simulink model "mrefrobotarm_previous_y_previous_u_previous_ref_cex_3b"  (R2018b)
settings: Solver=FixedStepAuto  StartTime=0.0  StopTime=20  RelTol=1e-3  AbsTol=1e-6
undefined symbols (not defined in the file or in its folder): cc, options
libraries: neural x462, simulink x2
(part 12 of 18)

== system mrefrobotarm_previous_y_previous_u_previous_ref_cex_3b/cex_m1/Layer 3/Delays 1 ==
  "p{3}" : Inport  PortDimensions=30
      mask Display: e = 0.06;c1 = [120 230 180]/255;c2 = ([120 230 180]+0)/(256+128);c3 = ([120 230 180]+128)/(256+128);patch([0 1 1 0],[0 0 1 1],c1);patch([0 1 1 1-e 1-e 0+e],[0 0 1 1-e 0+e 0+e],c2);patch([0 0 1 1-e 0+e 0+e],[0 1 1 1-e 1-e 0+e],c3);plot([0 1 1 0 0],[0 0 1 1 0]);
  mux : Mux  Inputs=1
      mask Display: e = 0.06;c1 = [120 150 230]/255;c2 = ([120 150 230]+0)/383;c3 = ([120 150 230]+128)/383;patch([0 1 1 0],[0 0 1 1],c1);patch([0 1 1 1-e 1-e 0+e],[0 0 1 1-e 0+e 0+e],c2);patch([0 0 1 1-e 0+e 0+e],[0 1 1 1-e 1-e 0+e],c3);plot([0 1 1 0 0],[0 0 1 1 0]);disp('Mux')
  "pd{3,2}" : Outport
      mask Display: e = 0.06;c1 = [120 230 180]/255;c2 = ([120 230 180]+0)/(256+128);c3 = ([120 230 180]+128)/(256+128);patch([0 1 1 0],[0 0 1 1],c1);patch([0 1 1 1-e 1-e 0+e],[0 0 1 1-e 0+e 0+e],c2);patch([0 0 1 1-e 0+e 0+e],[0 1 1 1-e 1-e 0+e],c3);plot([0 1 1 0 0],[0 0 1 1 0]);
  wires:
  "p{3}"/1 -> mux/1
  mux/1 -> "pd{3,2}"/1

== system mrefrobotarm_previous_y_previous_u_previous_ref_cex_3b/cex_m1/Layer 3/LW{3,2} ==
  "ad{3,2}" : Inport  PortDimensions=30
      mask Display: e = 0.06;c1 = [120 230 180]/255;c2 = ([120 230 180]+0)/(256+128);c3 = ([120 230 180]+128)/(256+128);patch([0 1 1 0],[0 0 1 1],c1);patch([0 1 1 1-e 1-e 0+e],[0 0 1 1-e 0+e 0+e],c2);patch([0 0 1 1-e 0+e 0+e],[0 1 1 1-e 1-e 0+e],c3);plot([0 1 1 0 0],[0 0 1 1 0]);
  "IW{3,2}(1,:)'" : Constant  Value=[0.0255900601227965381057050109347983379848301410675048828125;-0.2445332719523497233549136353758512996137142181396484375;0.2132234013283009488315400403735111467540264129638671875;-0.0515001036072283702171858976726070977747440338134765625;-0.19351367720373280345569355631596408784389495849609375;0.376109267327173701911391390240169130265712738037109375;0.0666749128615344577308832185735809616744518280029296875;-0.44077680308893107952172840668936260044574737548828125;-0.1774770708842355604328844265182851813733577728271484375;-0.054251675677824177934649441112924250774085521697998046875;0.407756480058180159620206950421561487019062042236328125;-0.11043832971419904886989371561867301352322101593017578125;-0.06656652324338363513334115850739181041717529296875;-0.309772314576237606242870015194057486951351165771484375;-0.2782579958208721837564780798857100307941436767578125;0.0014079282704737897634339471863995640887878835201263427734375;0.164750395979450681149813817683025263249874114990234375;0.03374371873575258973243506943617830984294414520263671875;-0.11697430223199604959471997744913096539676189422607421875;-0.377976875689660485324594674239051528275012969970703125;0.180234815360957700836053163584438152611255645751953125;0.049494338029175431736828016937579377554357051849365234375;-0.541724329864333054018743496271781623363494873046875;0.70957921545389057715880198884406127035617828369140625;-0.2236538006543592749242321815472678281366825103759765625;-0.0168625825253284934712727505257134907878935337066650390625;-0.061157151815638820246956441906149848364293575286865234375;0.0962999458349639014809184800469665788114070892333984375;-0.195422183072548050208894210300059057772159576416015625;0.469008564925858462135721538288635201752185821533203125]
      mask Display: e = 0.06;c1 = [120 150 230]/255;c2 = ([120 150 230]+0)/383;c3 = ([120 150 230]+128)/383;patch([0 1 1 0],[0 0 1 1],c1);patch([0 1 1 1-e 1-e 0+e],[0 0 1 1-e 0+e 0+e],c2);patch([0 0 1 1-e 0+e 0+e],[0 1 1 1-e 1-e 0+e],c3);plot([0 1 1 0 0],[0 0 1 1 0]);disp('weights');
  Mux : Mux  Inputs=1
      mask Display: e = 0.06;c1 = [120 150 230]/255;c2 = ([120 150 230]+0)/383;c3 = ([120 150 230]+128)/383;patch([0 1 1 0],[0 0 1 1],c1);patch([0 1 1 1-e 1-e 0+e],[0 0 1 1-e 0+e 0+e],c2);patch([0 0 1 1-e 0+e 0+e],[0 1 1 1-e 1-e 0+e],c3);plot([0 1 1 0 0],[0 0 1 1 0]);disp('Mux');
  dotprod1 : neural/Weight Functions/dotprod
  "lz{3,2}" : Outport
      mask Display: e = 0.06;c1 = [120 230 180]/255;c2 = ([120 230 180]+0)/(256+128);c3 = ([120 230 180]+128)/(256+128);patch([0 1 1 0],[0 0 1 1],c1);patch([0 1 1 1-e 1-e 0+e],[0 0 1 1-e 0+e 0+e],c2);patch([0 0 1 1-e 0+e 0+e],[0 1 1 1-e 1-e 0+e],c3);plot([0 1 1 0 0],[0 0 1 1 0]);
  wires:
  "IW{3,2}(1,:)'"/1 -> dotprod1/1
  "ad{3,2}"/1 -> dotprod1/2
  dotprod1/1 -> Mux/1
  Mux/1 -> "lz{3,2}"/1

== system mrefrobotarm_previous_y_previous_u_previous_ref_cex_3b/cex_m5/Layer 1/Delays 1 ==
  "p{1}" : Inport  PortDimensions=10
      mask Display: e = 0.06;c1 = [120 230 180]/255;c2 = ([120 230 180]+0)/(256+128);c3 = ([120 230 180]+128)/(256+128);patch([0 1 1 0],[0 0 1 1],c1);patch([0 1 1 1-e 1-e 0+e],[0 0 1 1-e 0+e 0+e],c2);patch([0 0 1 1-e 0+e 0+e],[0 1 1 1-e 1-e 0+e],c3);plot([0 1 1 0 0],[0 0 1 1 0]);
  mux : Mux  Inputs=1
      mask Display: e = 0.06;c1 = [120 150 230]/255;c2 = ([120 150 230]+0)/383;c3 = ([120 150 230]+128)/383;patch([0 1 1 0],[0 0 1 1],c1);patch([0 1 1 1-e 1-e 0+e],[0 0 1 1-e 0+e 0+e],c2);patch([0 0 1 1-e 0+e 0+e],[0 1 1 1-e 1-e 0+e],c3);plot([0 1 1 0 0],[0 0 1 1 0]);disp('Mux')
  "pd{1,1}" : Outport
      mask Display: e = 0.06;c1 = [120 230 180]/255;c2 = ([120 230 180]+0)/(256+128);c3 = ([120 230 180]+128)/(256+128);patch([0 1 1 0],[0 0 1 1],c1);patch([0 1 1 1-e 1-e 0+e],[0 0 1 1-e 0+e 0+e],c2);patch([0 0 1 1-e 0+e 0+e],[0 1 1 1-e 1-e 0+e],c3);plot([0 1 1 0 0],[0 0 1 1 0]);
  wires:
  "p{1}"/1 -> mux/1
  mux/1 -> "pd{1,1}"/1

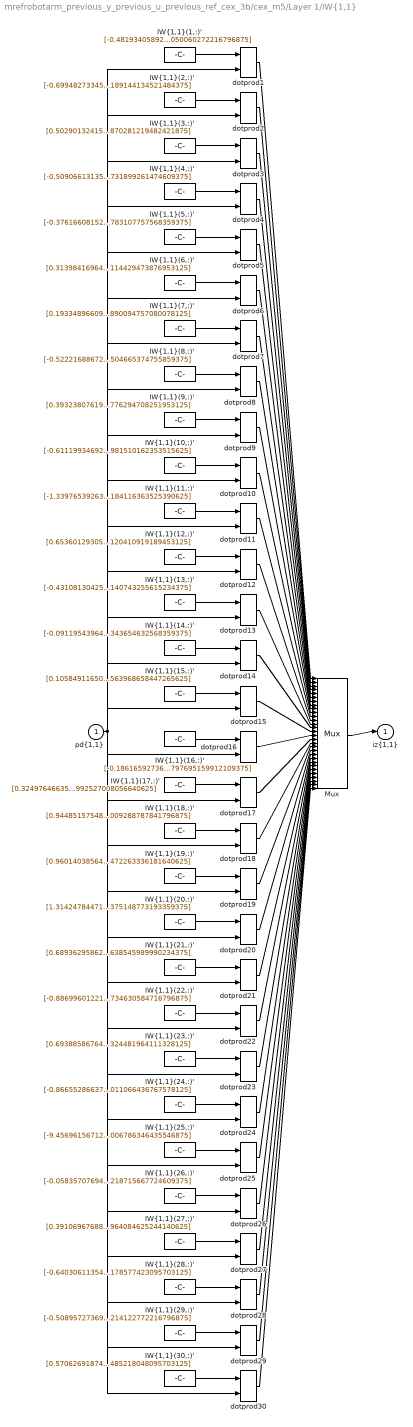
== system mrefrobotarm_previous_y_previous_u_previous_ref_cex_3b/cex_m5/Layer 1/IW{1,1} ==
  "pd{1,1}" : Inport  PortDimensions=10
      mask Display: e = 0.06;c1 = [120 230 180]/255;c2 = ([120 230 180]+0)/(256+128);c3 = ([120 230 180]+128)/(256+128);patch([0 1 1 0],[0 0 1 1],c1);patch([0 1 1 1-e 1-e 0+e],[0 0 1 1-e 0+e 0+e],c2);patch([0 0 1 1-e 0+e 0+e],[0 1 1 1-e 1-e 0+e],c3);plot([0 1 1 0 0],[0 0 1 1 0]);
  "IW{1,1}(1,:)'" : Constant  Value=[-0.481934058923276398278545684661366976797580718994140625;0.36530523689031058065523893674253486096858978271484375;-0.86926905168321899619598980279988609254360198974609375;-0.422931186541281534108094319890369661152362823486328125;0.50571230197535843586820192285813391208648681640625;-0.51255895275061913451963846455328166484832763671875;0.2023427088065134216154916657615103758871555328369140625;0.725871649925782680412567060557194054126739501953125;-0.16849060637558366249066921227495186030864715576171875;-0.205273588229551495754066081644850783050060272216796875]
      mask Display: e = 0.06;c1 = [120 150 230]/255;c2 = ([120 150 230]+0)/383;c3 = ([120 150 230]+128)/383;patch([0 1 1 0],[0 0 1 1],c1);patch([0 1 1 1-e 1-e 0+e],[0 0 1 1-e 0+e 0+e],c2);patch([0 0 1 1-e 0+e 0+e],[0 1 1 1-e 1-e 0+e],c3);plot([0 1 1 0 0],[0 0 1 1 0]);disp('Weights');
  "IW{1,1}(10,:)'" : Constant  Value=[-0.61119934692369726203509117112844251096248626708984375;0.70454804335546794558098326888284645974636077880859375;0.057135643818077175293268510358757339417934417724609375;0.89228683122494256707568638375960290431976318359375;-0.306202450351405086603762129016104154288768768310546875;-0.53945258802536877329458775420789606869220733642578125;0.413295177296751081730263877034303732216358184814453125;-0.86207965190394852950106496791704557836055755615234375;-0.77818630476135786100400082432315684854984283447265625;-0.9866456915733705645976669984520412981510162353515625]
      mask Display: e = 0.06;c1 = [120 150 230]/255;c2 = ([120 150 230]+0)/383;c3 = ([120 150 230]+128)/383;patch([0 1 1 0],[0 0 1 1],c1);patch([0 1 1 1-e 1-e 0+e],[0 0 1 1-e 0+e 0+e],c2);patch([0 0 1 1-e 0+e 0+e],[0 1 1 1-e 1-e 0+e],c3);plot([0 1 1 0 0],[0 0 1 1 0]);disp('Weights');
  "IW{1,1}(11,:)'" : Constant  Value=[-1.3397653926357528941792907062335871160030364990234375;2.106003584289421137754061419400386512279510498046875;-1.3291512443981907676260334483231417834758758544921875;0.462989686404331413083212964920676313340663909912109375;-6.6943247779396433116971820709295570850372314453125;0.1574200960671499893717140139415278099477291107177734375;3.689170060642462001254671122296713292598724365234375;0.455374095081902907633519816954503767192363739013671875;-3.653332928797798473397051566280424594879150390625;-2.427542355801075135701694307499565184116363525390625]
      mask Display: e = 0.06;c1 = [120 150 230]/255;c2 = ([120 150 230]+0)/383;c3 = ([120 150 230]+128)/383;patch([0 1 1 0],[0 0 1 1],c1);patch([0 1 1 1-e 1-e 0+e],[0 0 1 1-e 0+e 0+e],c2);patch([0 0 1 1-e 0+e 0+e],[0 1 1 1-e 1-e 0+e],c3);plot([0 1 1 0 0],[0 0 1 1 0]);disp('Weights');
  "IW{1,1}(12,:)'" : Constant  Value=[0.6536012930577299595569229495595209300518035888671875;-0.9465981615866529974567811223096214234828948974609375;0.68180864552264408562365360921830870211124420166015625;0.95131511966430759574819830959313549101352691650390625;-0.63476802573249646588493533272412605583667755126953125;0.51713095973796685544954243596293963491916656494140625;-0.429683896760812700232889937979052774608135223388671875;0.27656440745969657069025515738758258521556854248046875;-0.81519572662588746236878023410099558532238006591796875;-0.043845142330680049458369040848992881365120410919189453125]
      mask Display: e = 0.06;c1 = [120 150 230]/255;c2 = ([120 150 230]+0)/383;c3 = ([120 150 230]+128)/383;patch([0 1 1 0],[0 0 1 1],c1);patch([0 1 1 1-e 1-e 0+e],[0 0 1 1-e 0+e 0+e],c2);patch([0 0 1 1-e 0+e 0+e],[0 1 1 1-e 1-e 0+e],c3);plot([0 1 1 0 0],[0 0 1 1 0]);disp('Weights');
  "IW{1,1}(13,:)'" : Constant  Value=[-0.431081304259618713903279285659664310514926910400390625;-0.73698073178504996949556016261340118944644927978515625;0.83120003960029098521999912918545305728912353515625;-0.7962063900043505615400363240041770040988922119140625;0.72949447017511992452654112639720551669597625732421875;-0.1515154460804853109312517744911019690334796905517578125;-0.396818838713428212461309385616914369165897369384765625;-0.2184960021029560828242921388664399273693561553955078125;1.193590255334305627599178478703834116458892822265625;0.041743865980058601772295645560006960295140743255615234375]
      mask Display: e = 0.06;c1 = [120 150 230]/255;c2 = ([120 150 230]+0)/383;c3 = ([120 150 230]+128)/383;patch([0 1 1 0],[0 0 1 1],c1);patch([0 1 1 1-e 1-e 0+e],[0 0 1 1-e 0+e 0+e],c2);patch([0 0 1 1-e 0+e 0+e],[0 1 1 1-e 1-e 0+e],c3);plot([0 1 1 0 0],[0 0 1 1 0]);disp('Weights');
  "IW{1,1}(14,:)'" : Constant  Value=[-0.091195439649284448790922397165559232234954833984375;-0.99484158954128909524428081567748449742794036865234375;0.87901205546453586858746120924479328095912933349609375;0.83500778529833163954521069172187708318233489990234375;0.1644769476026444465777132108996738679707050323486328125;0.299859204492049169488154802820645272731781005859375;-0.675293267990959567015352149610407650470733642578125;-0.6724048304577507906287792138755321502685546875;-0.488273399712188915788857457300764508545398712158203125;0.7939591905605707378157376297167502343654632568359375]
      mask Display: e = 0.06;c1 = [120 150 230]/255;c2 = ([120 150 230]+0)/383;c3 = ([120 150 230]+128)/383;patch([0 1 1 0],[0 0 1 1],c1);patch([0 1 1 1-e 1-e 0+e],[0 0 1 1-e 0+e 0+e],c2);patch([0 0 1 1-e 0+e 0+e],[0 1 1 1-e 1-e 0+e],c3);plot([0 1 1 0 0],[0 0 1 1 0]);disp('Weights');
  "IW{1,1}(15,:)'" : Constant  Value=[0.1058491165092696750793521687228349037468433380126953125;-1.0597129577604322836492656279006041586399078369140625;-0.08565748424271346639358171159983612596988677978515625;-0.65493557690493509060303267688141204416751861572265625;0.5592429102064613299916118194232694804668426513671875;0.866348192195701027884524592082016170024871826171875;-0.8557577843621329005685538504621945321559906005859375;-0.145254205489326826405971360145485959947109222412109375;1.0167202066568445939509501840802840888500213623046875;-0.41676857755055696230783723876811563968658447265625]
      mask Display: e = 0.06;c1 = [120 150 230]/255;c2 = ([120 150 230]+0)/383;c3 = ([120 150 230]+128)/383;patch([0 1 1 0],[0 0 1 1],c1);patch([0 1 1 1-e 1-e 0+e],[0 0 1 1-e 0+e 0+e],c2);patch([0 0 1 1-e 0+e 0+e],[0 1 1 1-e 1-e 0+e],c3);plot([0 1 1 0 0],[0 0 1 1 0]);disp('Weights');
  "IW{1,1}(16,:)'" : Constant  Value=[-0.18616592736444814715213169620255939662456512451171875;0.6141017141754818720045250302064232528209686279296875;0.77741432437768842600434027190203778445720672607421875;0.450158418931855208722225825113127939403057098388671875;-0.7541351529836557432417976087890565395355224609375;-0.67449785750865565159273273820872418582439422607421875;-0.48980390262855932892449573046178556978702545166015625;0.72765822408069713578271375808981247246265411376953125;-0.9126600152434176660420916959992609918117523193359375;-0.1885993036556745661158629445708356797695159912109375]
      mask Display: e = 0.06;c1 = [120 150 230]/255;c2 = ([120 150 230]+0)/383;c3 = ([120 150 230]+128)/383;patch([0 1 1 0],[0 0 1 1],c1);patch([0 1 1 1-e 1-e 0+e],[0 0 1 1-e 0+e 0+e],c2);patch([0 0 1 1-e 0+e 0+e],[0 1 1 1-e 1-e 0+e],c3);plot([0 1 1 0 0],[0 0 1 1 0]);disp('Weights');
  "IW{1,1}(17,:)'" : Constant  Value=[0.32497646635307997353692144315573386847972869873046875;-1.058499332324482455902625588350929319858551025390625;0.56967924448973839002263730435515753924846649169921875;0.1831651507289188407501256961040780879557132720947265625;-0.84754674951697983598108976366347633302211761474609375;0.5389689674319024792481513941311277449131011962890625;-0.39284692552225586315017835659091360867023468017578125;-0.26814251044309200810999982422799803316593170166015625;1.2499036209033544952973215913516469299793243408203125;0.0652351666789356132714061686783679760992527008056640625]
      mask Display: e = 0.06;c1 = [120 150 230]/255;c2 = ([120 150 230]+0)/383;c3 = ([120 150 230]+128)/383;patch([0 1 1 0],[0 0 1 1],c1);patch([0 1 1 1-e 1-e 0+e],[0 0 1 1-e 0+e 0+e],c2);patch([0 0 1 1-e 0+e 0+e],[0 1 1 1-e 1-e 0+e],c3);plot([0 1 1 0 0],[0 0 1 1 0]);disp('Weights');
  "IW{1,1}(18,:)'" : Constant  Value=[0.944851575482778205383738168166019022464752197265625;0.40233748698709603797141198811004869639873504638671875;0.296700025402451827982730492294649593532085418701171875;-0.5705011227590153222166691193706355988979339599609375;0.62399684535928179318631237038061954081058502197265625;-0.666993826985459836720337989390827715396881103515625;1.319033892293299370379600077285431325435638427734375;-0.2355276087914129623523962209219462238252162933349609375;-0.822732979392644114824406642583198845386505126953125;0.3973861416747854757858249286073260009288787841796875]
      mask Display: e = 0.06;c1 = [120 150 230]/255;c2 = ([120 150 230]+0)/383;c3 = ([120 150 230]+128)/383;patch([0 1 1 0],[0 0 1 1],c1);patch([0 1 1 1-e 1-e 0+e],[0 0 1 1-e 0+e 0+e],c2);patch([0 0 1 1-e 0+e 0+e],[0 1 1 1-e 1-e 0+e],c3);plot([0 1 1 0 0],[0 0 1 1 0]);disp('Weights');
  "IW{1,1}(19,:)'" : Constant  Value=[0.9601403856428356586860672905459068715572357177734375;0.420991330967579735489181302909855730831623077392578125;-0.295265802335514582210862499778158962726593017578125;0.16617442563824358359170219046063721179962158203125;-0.00964743545283248786492702464556714403443038463592529296875;-0.5598062825266023612158505784464068710803985595703125;-0.79565186921215858006917187594808638095855712890625;0.2119124317163829374077721467983792535960674285888671875;1.4074992486424793280974654408055357635021209716796875;0.5302701993277880720967232264229096472263336181640625]
      mask Display: e = 0.06;c1 = [120 150 230]/255;c2 = ([120 150 230]+0)/383;c3 = ([120 150 230]+128)/383;patch([0 1 1 0],[0 0 1 1],c1);patch([0 1 1 1-e 1-e 0+e],[0 0 1 1-e 0+e 0+e],c2);patch([0 0 1 1-e 0+e 0+e],[0 1 1 1-e 1-e 0+e],c3);plot([0 1 1 0 0],[0 0 1 1 0]);disp('Weights');
  "IW{1,1}(2,:)'" : Constant  Value=[-0.699482733452999827505891516921110451221466064453125;-0.52887549308012282711644047594745643436908721923828125;0.84729521568959154098621411321801133453845977783203125;0.908000823746515361989395387354306876659393310546875;-0.156414778112398789033932189340703189373016357421875;-0.76080952924288303140798461754457093775272369384765625;0.19992807142769375428059674959513358771800994873046875;-0.054254242839367916584336626328877173364162445068359375;2.198635801063346661976538598537445068359375;1.8375597568026778017014066790579818189144134521484375]
      mask Display: e = 0.06;c1 = [120 150 230]/255;c2 = ([120 150 230]+0)/383;c3 = ([120 150 230]+128)/383;patch([0 1 1 0],[0 0 1 1],c1);patch([0 1 1 1-e 1-e 0+e],[0 0 1 1-e 0+e 0+e],c2);patch([0 0 1 1-e 0+e 0+e],[0 1 1 1-e 1-e 0+e],c3);plot([0 1 1 0 0],[0 0 1 1 0]);disp('Weights');
  "IW{1,1}(20,:)'" : Constant  Value=[1.3142478447186667356305633802548982203006744384765625;0.8981046381155268765184018775471486151218414306640625;-0.18627134029377534485405476516461931169033050537109375;-0.82621028255460993161563010289683006703853607177734375;-0.278152135018808588373673273963504470884799957275390625;0.77412259718377163242308824919746257364749908447265625;0.154756053944371474440089286872535012662410736083984375;0.1254386379596720557660916028908104635775089263916015625;-0.03881968560856623173815904692673939280211925506591796875;-0.7116181981742639717225529238930903375148773193359375]
      mask Display: e = 0.06;c1 = [120 150 230]/255;c2 = ([120 150 230]+0)/383;c3 = ([120 150 230]+128)/383;patch([0 1 1 0],[0 0 1 1],c1);patch([0 1 1 1-e 1-e 0+e],[0 0 1 1-e 0+e 0+e],c2);patch([0 0 1 1-e 0+e 0+e],[0 1 1 1-e 1-e 0+e],c3);plot([0 1 1 0 0],[0 0 1 1 0]);disp('Weights');
  "IW{1,1}(21,:)'" : Constant  Value=[0.68936295862615881713253429552423767745494842529296875;-0.82313775715762760309957002391456626355648040771484375;0.8270386896732215831207213341258466243743896484375;-0.26689409148944476246612111935974098742008209228515625;0.43046182480710359907760675923782400786876678466796875;-0.78175408480938612942878762623877264559268951416015625;-0.6696365368601402412451761847478337585926055908203125;0.0622811083876329274477967601342243142426013946533203125;0.71519232793105647072451347412425093352794647216796875;0.40600619794918324512167373541160486638545989990234375]
      mask Display: e = 0.06;c1 = [120 150 230]/255;c2 = ([120 150 230]+0)/383;c3 = ([120 150 230]+128)/383;patch([0 1 1 0],[0 0 1 1],c1);patch([0 1 1 1-e 1-e 0+e],[0 0 1 1-e 0+e 0+e],c2);patch([0 0 1 1-e 0+e 0+e],[0 1 1 1-e 1-e 0+e],c3);plot([0 1 1 0 0],[0 0 1 1 0]);disp('Weights');
  "IW{1,1}(22,:)'" : Constant  Value=[-0.8869960122165967408847109254566021263599395751953125;0.89520437559754773015896489596343599259853363037109375;0.0240188990354666571935826624439869192428886890411376953125;-0.458839502593588743906138915917836129665374755859375;0.19460753710154232720697109471075236797332763671875;0.81439676886340517381057679813238792121410369873046875;-0.14772142147908728926353205679333768784999847412109375;-0.8800421927112231923473473216290585696697235107421875;-0.39143880357146632054110568788019008934497833251953125;-0.194415229870990191596291651876526884734630584716796875]
      mask Display: e = 0.06;c1 = [120 150 230]/255;c2 = ([120 150 230]+0)/383;c3 = ([120 150 230]+128)/383;patch([0 1 1 0],[0 0 1 1],c1);patch([0 1 1 1-e 1-e 0+e],[0 0 1 1-e 0+e 0+e],c2);patch([0 0 1 1-e 0+e 0+e],[0 1 1 1-e 1-e 0+e],c3);plot([0 1 1 0 0],[0 0 1 1 0]);disp('Weights');
  "IW{1,1}(23,:)'" : Constant  Value=[0.69388586764422310881883504407596774399280548095703125;-0.852497148226928569414440062246285378932952880859375;0.025772392646516817382718045337242074310779571533203125;-0.458625523961370074044197053808602504432201385498046875;-0.51130637160668424012754940122249536216259002685546875;-0.008827476680515589091413630740134976804256439208984375;0.751314296642477952303806887357495725154876708984375;0.92074387932284318392106570172472856938838958740234375;0.04196420456835599221978583273084950633347034454345703125;0.8451662610983448065127277004648931324481964111328125]
      mask Display: e = 0.06;c1 = [120 150 230]/255;c2 = ([120 150 230]+0)/383;c3 = ([120 150 230]+128)/383;patch([0 1 1 0],[0 0 1 1],c1);patch([0 1 1 1-e 1-e 0+e],[0 0 1 1-e 0+e 0+e],c2);patch([0 0 1 1-e 0+e 0+e],[0 1 1 1-e 1-e 0+e],c3);plot([0 1 1 0 0],[0 0 1 1 0]);disp('Weights');
  "IW{1,1}(24,:)'" : Constant  Value=[-0.8665528663708557122191677990485914051532745361328125;-0.3082624255230459464627301713335327804088592529296875;0.402126549567523416950365344746387563645839691162109375;0.69030442209237519168851804352016188204288482666015625;0.8024336892819394773113117480534128844738006591796875;0.154259749947727897723126488926936872303485870361328125;-1.2495973770855293150106035682256333529949188232421875;-0.2420454425610247539690789153610239736735820770263671875;0.31995666039149328607749112052260898053646087646484375;-0.12310643949809270403239480629054014571011066436767578125]
      mask Display: e = 0.06;c1 = [120 150 230]/255;c2 = ([120 150 230]+0)/383;c3 = ([120 150 230]+128)/383;patch([0 1 1 0],[0 0 1 1],c1);patch([0 1 1 1-e 1-e 0+e],[0 0 1 1-e 0+e 0+e],c2);patch([0 0 1 1-e 0+e 0+e],[0 1 1 1-e 1-e 0+e],c3);plot([0 1 1 0 0],[0 0 1 1 0]);disp('Weights');
  "IW{1,1}(25,:)'" : Constant  Value=[-9.456961567121421552428728318773210048675537109375;10.1594158142121937515867102774791419506072998046875;0.712745074701544023554333762149326503276824951171875;-0.71340225812910118552423455184907652437686920166015625;1.6857423854082387304487156143295578658580780029296875;-3.544430859880379092174962352146394550800323486328125;13.958092206597338957863030373118817806243896484375;-12.02152129868098739962078980170190334320068359375;3.536895982920345904432224415359087288379669189453125;0.526923484683730958266778543475084006786346435546875]
      mask Display: e = 0.06;c1 = [120 150 230]/255;c2 = ([120 150 230]+0)/383;c3 = ([120 150 230]+128)/383;patch([0 1 1 0],[0 0 1 1],c1);patch([0 1 1 1-e 1-e 0+e],[0 0 1 1-e 0+e 0+e],c2);patch([0 0 1 1-e 0+e 0+e],[0 1 1 1-e 1-e 0+e],c3);plot([0 1 1 0 0],[0 0 1 1 0]);disp('Weights');
  "IW{1,1}(26,:)'" : Constant  Value=[-0.058357076945515500010497333960302057676017284393310546875;0.290966944383173053978453026502393186092376708984375;0.7700729005838369278791333272238261997699737548828125;0.60486513303375233352454642954398877918720245361328125;0.308320026178229678048836603920790366828441619873046875;-0.90990786985333471648118575103580951690673828125;0.9558615914645567368523870754870586097240447998046875;-0.66295614739857622321750341143342666327953338623046875;-0.274789838020543075725043991042184643447399139404296875;0.205342551049631116821814202921814285218715667724609375]
      mask Display: e = 0.06;c1 = [120 150 230]/255;c2 = ([120 150 230]+0)/383;c3 = ([120 150 230]+128)/383;patch([0 1 1 0],[0 0 1 1],c1);patch([0 1 1 1-e 1-e 0+e],[0 0 1 1-e 0+e 0+e],c2);patch([0 0 1 1-e 0+e 0+e],[0 1 1 1-e 1-e 0+e],c3);plot([0 1 1 0 0],[0 0 1 1 0]);disp('Weights');
  "IW{1,1}(27,:)'" : Constant  Value=[0.391069676883912864528980435352423228323459625244140625;-0.369224399691742422024987035911181010305881500244140625;0.2044572544139468261992220732281566597521305084228515625;0.55234686807135513486599620591732673346996307373046875;0.44198555383566695553554382058791816234588623046875;-1.0840323746493074619223762056208215653896331787109375;-0.49123059812482317010307042437489144504070281982421875;0.7599744739031313311983240055269561707973480224609375;-0.54228025557021342084595971755334176123142242431640625;-1.4175296458265977950219394188025034964084625244140625]
      mask Display: e = 0.06;c1 = [120 150 230]/255;c2 = ([120 150 230]+0)/383;c3 = ([120 150 230]+128)/383;patch([0 1 1 0],[0 0 1 1],c1);patch([0 1 1 1-e 1-e 0+e],[0 0 1 1-e 0+e 0+e],c2);patch([0 0 1 1-e 0+e 0+e],[0 1 1 1-e 1-e 0+e],c3);plot([0 1 1 0 0],[0 0 1 1 0]);disp('Weights');
  "IW{1,1}(28,:)'" : Constant  Value=[-0.64030611354245869915047251197393052279949188232421875;-0.1813249666234290902178116766663151793181896209716796875;-1.1488699140949929500266080140136182308197021484375;1.35511253789927454960206887335516512393951416015625;0.411547285591023104256436226933146826922893524169921875;-0.76055420298351805730163732732762582600116729736328125;0.48129301813141889265779127526911906898021697998046875;-1.3260502947565624420889207613072358071804046630859375;0.9713869907910479550849913721322081983089447021484375;-0.277689358717902845530289823727798648178577423095703125]
      mask Display: e = 0.06;c1 = [120 150 230]/255;c2 = ([120 150 230]+0)/383;c3 = ([120 150 230]+128)/383;patch([0 1 1 0],[0 0 1 1],c1);patch([0 1 1 1-e 1-e 0+e],[0 0 1 1-e 0+e 0+e],c2);patch([0 0 1 1-e 0+e 0+e],[0 1 1 1-e 1-e 0+e],c3);plot([0 1 1 0 0],[0 0 1 1 0]);disp('Weights');
  "IW{1,1}(29,:)'" : Constant  Value=[-0.50895727369880627843912179741892032325267791748046875;0.67215894066086623315214865215239115059375762939453125;0.15067344077122246659428128623403608798980712890625;-1.236765974242786114700720645487308502197265625;0.2057155400994366833966608965056366287171840667724609375;0.934248659264587555384196093655191361904144287109375;-0.27181155293088909985499412869103252887725830078125;-0.2282395717535073143000801110247266478836536407470703125;0.11123914324454575730527494670241139829158782958984375;-0.972841022608480709976674916106276214122772216796875]
      mask Display: e = 0.06;c1 = [120 150 230]/255;c2 = ([120 150 230]+0)/383;c3 = ([120 150 230]+128)/383;patch([0 1 1 0],[0 0 1 1],c1);patch([0 1 1 1-e 1-e 0+e],[0 0 1 1-e 0+e 0+e],c2);patch([0 0 1 1-e 0+e 0+e],[0 1 1 1-e 1-e 0+e],c3);plot([0 1 1 0 0],[0 0 1 1 0]);disp('Weights');
  "IW{1,1}(3,:)'" : Constant  Value=[0.5029013241536066658454728894867002964019775390625;0.50276940705494421735011201235465705394744873046875;-0.0239780897556748084920030805733404122292995452880859375;-0.7624437289848560173055602717795409262180328369140625;-1.1806890530636422464993984249304048717021942138671875;0.38987192849709384478984475208562798798084259033203125;-0.02187079195207548842905254105062340386211872100830078125;0.17376337641484795870638890846748836338520050048828125;0.14589582823772195840916765519068576395511627197265625;2.586770563285153201604771311394870281219482421875]
      mask Display: e = 0.06;c1 = [120 150 230]/255;c2 = ([120 150 230]+0)/383;c3 = ([120 150 230]+128)/383;patch([0 1 1 0],[0 0 1 1],c1);patch([0 1 1 1-e 1-e 0+e],[0 0 1 1-e 0+e 0+e],c2);patch([0 0 1 1-e 0+e 0+e],[0 1 1 1-e 1-e 0+e],c3);plot([0 1 1 0 0],[0 0 1 1 0]);disp('Weights');
  "IW{1,1}(30,:)'" : Constant  Value=[0.5706269187427828182279654356534592807292938232421875;-0.57824573232220888296950533913332037627696990966796875;-0.3610888283156106215443514884100295603275299072265625;-0.41774248508584721495395797319361008703708648681640625;0.490831694763102621692496541072614490985870361328125;1.0738201332865784376480178252677433192729949951171875;1.0357549947689872471556782329571433365345001220703125;-0.393416337831026974303227916607283987104892730712890625;0.5156947722138156553484122923691757023334503173828125;-0.1880426242408612946821477862613392062485218048095703125]
      mask Display: e = 0.06;c1 = [120 150 230]/255;c2 = ([120 150 230]+0)/383;c3 = ([120 150 230]+128)/383;patch([0 1 1 0],[0 0 1 1],c1);patch([0 1 1 1-e 1-e 0+e],[0 0 1 1-e 0+e 0+e],c2);patch([0 0 1 1-e 0+e 0+e],[0 1 1 1-e 1-e 0+e],c3);plot([0 1 1 0 0],[0 0 1 1 0]);disp('Weights');
  "IW{1,1}(4,:)'" : Constant  Value=[-0.5090661313546192001666668147663585841655731201171875;0.38409125075119943115709020275971852242946624755859375;-0.542303975129727167114879193832166492938995361328125;0.723642128782074234294441339443437755107879638671875;-0.2034072493422434124710207470343448221683502197265625;0.50221523201678108794254740132601000368595123291015625;1.0707368137493225024314824622706510126590728759765625;-0.09960789021163511669509915691378409974277019500732421875;-0.76909992741888277834050313686020672321319580078125;-0.73801919165111140586077453917823731899261474609375]
      mask Display: e = 0.06;c1 = [120 150 230]/255;c2 = ([120 150 230]+0)/383;c3 = ([120 150 230]+128)/383;patch([0 1 1 0],[0 0 1 1],c1);patch([0 1 1 1-e 1-e 0+e],[0 0 1 1-e 0+e 0+e],c2);patch([0 0 1 1-e 0+e 0+e],[0 1 1 1-e 1-e 0+e],c3);plot([0 1 1 0 0],[0 0 1 1 0]);disp('Weights');
  "IW{1,1}(5,:)'" : Constant  Value=[-0.37616608152094632711026633842266164720058441162109375;-0.08595969067818189091045866234708228148519992828369140625;0.64491430020224782548865505305002443492412567138671875;-0.1468342956231186435811508772530942223966121673583984375;-0.77327774905845336750331853181705810129642486572265625;0.95540889613754753639796035713516175746917724609375;0.3105698141414461321829776352387852966785430908203125;0.56044219953083718177566652229870669543743133544921875;-0.47269827268512909501652075050515122711658477783203125;0.481133559231257945665305442162207327783107757568359375]
      mask Display: e = 0.06;c1 = [120 150 230]/255;c2 = ([120 150 230]+0)/383;c3 = ([120 150 230]+128)/383;patch([0 1 1 0],[0 0 1 1],c1);patch([0 1 1 1-e 1-e 0+e],[0 0 1 1-e 0+e 0+e],c2);patch([0 0 1 1-e 0+e 0+e],[0 1 1 1-e 1-e 0+e],c3);plot([0 1 1 0 0],[0 0 1 1 0]);disp('Weights');
  "IW{1,1}(6,:)'" : Constant  Value=[0.3139841696478213872723017630050890147686004638671875;-0.72960289215258866679647553610266186296939849853515625;0.41593945028168410882329908417887054383754730224609375;-0.80492549266935575769110755572910420596599578857421875;0.63039551400000448655447371493210084736347198486328125;-0.7730789039616876578975279699079692363739013671875;-0.25019703736153064976832638421910814940929412841796875;0.7098637487107655186235888322698883712291717529296875;-1.653242639930166291151181212626397609710693359375;0.0263862065668849510302607086487114429473876953125]
      mask Display: e = 0.06;c1 = [120 150 230]/255;c2 = ([120 150 230]+0)/383;c3 = ([120 150 230]+128)/383;patch([0 1 1 0],[0 0 1 1],c1);patch([0 1 1 1-e 1-e 0+e],[0 0 1 1-e 0+e 0+e],c2);patch([0 0 1 1-e 0+e 0+e],[0 1 1 1-e 1-e 0+e],c3);plot([0 1 1 0 0],[0 0 1 1 0]);disp('Weights');
  "IW{1,1}(7,:)'" : Constant  Value=[0.1933489660931838327595500004463247023522853851318359375;0.9713519291773289321412221397622488439083099365234375;0.11590498675470757572458779804946971125900745391845703125;-0.6358705065441221382371850268100388348102569580078125;-0.35617986877142182589039975937339477241039276123046875;-0.6662549486376454499492183458642102777957916259765625;-0.655224049966256938404285392607562243938446044921875;-0.25588616037893341381703748993459157645702362060546875;-1.0097655264731084656659731990657746791839599609375;-0.62485294692444448561019498811219818890094757080078125]
      mask Display: e = 0.06;c1 = [120 150 230]/255;c2 = ([120 150 230]+0)/383;c3 = ([120 150 230]+128)/383;patch([0 1 1 0],[0 0 1 1],c1);patch([0 1 1 1-e 1-e 0+e],[0 0 1 1-e 0+e 0+e],c2);patch([0 0 1 1-e 0+e 0+e],[0 1 1 1-e 1-e 0+e],c3);plot([0 1 1 0 0],[0 0 1 1 0]);disp('Weights');
  "IW{1,1}(8,:)'" : Constant  Value=[-0.52221688672633070904538499235059134662151336669921875;0.5108610597035536660115440099616535007953643798828125;-0.77174690291767245042819922673515975475311279296875;-0.3763500782301407721064379074960015714168548583984375;0.3932913904308394936748527470626868307590484619140625;-0.21801111213087820406286709840060211718082427978515625;0.28269749300520607970810260667349211871623992919921875;0.8790627462558713300921908739837817847728729248046875;-0.85675911437050034091811312464415095746517181396484375;0.9091764853771504562018890283070504665374755859375]
      mask Display: e = 0.06;c1 = [120 150 230]/255;c2 = ([120 150 230]+0)/383;c3 = ([120 150 230]+128)/383;patch([0 1 1 0],[0 0 1 1],c1);patch([0 1 1 1-e 1-e 0+e],[0 0 1 1-e 0+e 0+e],c2);patch([0 0 1 1-e 0+e 0+e],[0 1 1 1-e 1-e 0+e],c3);plot([0 1 1 0 0],[0 0 1 1 0]);disp('Weights');
  "IW{1,1}(9,:)'" : Constant  Value=[0.393238076195151553537954214334604330360889434814453125;0.53951562895778248929445908288471400737762451171875;-0.7150070155681682582127223213319666683673858642578125;-0.324490161291762391204684945478220470249652862548828125;-0.41795059520567134914159623804152943193912506103515625;1.0636424093396288359514301191666163504123687744140625;0.88419732209727630589668478933162987232208251953125;0.0645062139885363705626986075003514997661113739013671875;-1.111768722669127296143187777488492429256439208984375;-1.5143656587610199171223257508245296776294708251953125]
      mask Display: e = 0.06;c1 = [120 150 230]/255;c2 = ([120 150 230]+0)/383;c3 = ([120 150 230]+128)/383;patch([0 1 1 0],[0 0 1 1],c1);patch([0 1 1 1-e 1-e 0+e],[0 0 1 1-e 0+e 0+e],c2);patch([0 0 1 1-e 0+e 0+e],[0 1 1 1-e 1-e 0+e],c3);plot([0 1 1 0 0],[0 0 1 1 0]);disp('Weights');
  Mux : Mux  Inputs=30
      mask Display: e = 0.06;c1 = [120 150 230]/255;c2 = ([120 150 230]+0)/383;c3 = ([120 150 230]+128)/383;patch([0 1 1 0],[0 0 1 1],c1);patch([0 1 1 1-e 1-e 0+e],[0 0 1 1-e 0+e 0+e],c2);patch([0 0 1 1-e 0+e 0+e],[0 1 1 1-e 1-e 0+e],c3);plot([0 1 1 0 0],[0 0 1 1 0]);disp('Mux');
  dotprod{1..30} (30 alike) : neural/Weight Functions/dotprod
  "iz{1,1}" : Outport
      mask Display: e = 0.06;c1 = [120 230 180]/255;c2 = ([120 230 180]+0)/(256+128);c3 = ([120 230 180]+128)/(256+128);patch([0 1 1 0],[0 0 1 1],c1);patch([0 1 1 1-e 1-e 0+e],[0 0 1 1-e 0+e 0+e],c2);patch([0 0 1 1-e 0+e 0+e],[0 1 1 1-e 1-e 0+e],c3);plot([0 1 1 0 0],[0 0 1 1 0]);
  wires:
  "IW{1,1}(1,:)'"/1 -> dotprod1/1
  "pd{1,1}"/1 -> dotprod1/2, dotprod2/2, dotprod3/2, dotprod4/2, dotprod5/2, dotprod6/2, dotprod7/2, dotprod8/2, dotprod9/2, dotprod10/2, dotprod11/2, dotprod12/2, dotprod13/2, dotprod14/2, dotprod15/2, dotprod16/2, dotprod17/2, dotprod18/2, dotprod19/2, dotprod20/2, dotprod21/2, dotprod22/2, dotprod23/2, dotprod24/2, dotprod25/2, dotprod26/2, dotprod27/2, dotprod28/2, dotprod29/2, dotprod30/2
  dotprod1/1 -> Mux/1
  "IW{1,1}(2,:)'"/1 -> dotprod2/1
  dotprod2/1 -> Mux/2
  "IW{1,1}(3,:)'"/1 -> dotprod3/1
  dotprod3/1 -> Mux/3
  "IW{1,1}(4,:)'"/1 -> dotprod4/1
  dotprod4/1 -> Mux/4
  "IW{1,1}(5,:)'"/1 -> dotprod5/1
  dotprod5/1 -> Mux/5
  "IW{1,1}(6,:)'"/1 -> dotprod6/1
  dotprod6/1 -> Mux/6
  "IW{1,1}(7,:)'"/1 -> dotprod7/1
  dotprod7/1 -> Mux/7
  "IW{1,1}(8,:)'"/1 -> dotprod8/1
  dotprod8/1 -> Mux/8
  "IW{1,1}(9,:)'"/1 -> dotprod9/1
  dotprod9/1 -> Mux/9
  "IW{1,1}(10,:)'"/1 -> dotprod10/1
  dotprod10/1 -> Mux/10
  "IW{1,1}(11,:)'"/1 -> dotprod11/1
  dotprod11/1 -> Mux/11
  "IW{1,1}(12,:)'"/1 -> dotprod12/1
  dotprod12/1 -> Mux/12
  "IW{1,1}(13,:)'"/1 -> dotprod13/1
  dotprod13/1 -> Mux/13
  "IW{1,1}(14,:)'"/1 -> dotprod14/1
  dotprod14/1 -> Mux/14
  "IW{1,1}(15,:)'"/1 -> dotprod15/1
  dotprod15/1 -> Mux/15
  "IW{1,1}(16,:)'"/1 -> dotprod16/1
  dotprod16/1 -> Mux/16
  "IW{1,1}(17,:)'"/1 -> dotprod17/1
  dotprod17/1 -> Mux/17
  "IW{1,1}(18,:)'"/1 -> dotprod18/1
  dotprod18/1 -> Mux/18
  "IW{1,1}(19,:)'"/1 -> dotprod19/1
  dotprod19/1 -> Mux/19
  "IW{1,1}(20,:)'"/1 -> dotprod20/1
  dotprod20/1 -> Mux/20
  "IW{1,1}(21,:)'"/1 -> dotprod21/1
  dotprod21/1 -> Mux/21
  "IW{1,1}(22,:)'"/1 -> dotprod22/1
  dotprod22/1 -> Mux/22
  "IW{1,1}(23,:)'"/1 -> dotprod23/1
  dotprod23/1 -> Mux/23
  "IW{1,1}(24,:)'"/1 -> dotprod24/1
  dotprod24/1 -> Mux/24
  "IW{1,1}(25,:)'"/1 -> dotprod25/1
  dotprod25/1 -> Mux/25
  "IW{1,1}(26,:)'"/1 -> dotprod26/1
  dotprod26/1 -> Mux/26
  "IW{1,1}(27,:)'"/1 -> dotprod27/1
  dotprod27/1 -> Mux/27
  "IW{1,1}(28,:)'"/1 -> dotprod28/1
  dotprod28/1 -> Mux/28
  "IW{1,1}(29,:)'"/1 -> dotprod29/1
  dotprod29/1 -> Mux/29
  "IW{1,1}(30,:)'"/1 -> dotprod30/1
  dotprod30/1 -> Mux/30
  Mux/1 -> "iz{1,1}"/1

== system mrefrobotarm_previous_y_previous_u_previous_ref_cex_3b/cex_m5/Layer 2/Delays 1 ==
  "p{2}" : Inport  PortDimensions=30
      mask Display: e = 0.06;c1 = [120 230 180]/255;c2 = ([120 230 180]+0)/(256+128);c3 = ([120 230 180]+128)/(256+128);patch([0 1 1 0],[0 0 1 1],c1);patch([0 1 1 1-e 1-e 0+e],[0 0 1 1-e 0+e 0+e],c2);patch([0 0 1 1-e 0+e 0+e],[0 1 1 1-e 1-e 0+e],c3);plot([0 1 1 0 0],[0 0 1 1 0]);
  mux : Mux  Inputs=1
      mask Display: e = 0.06;c1 = [120 150 230]/255;c2 = ([120 150 230]+0)/383;c3 = ([120 150 230]+128)/383;patch([0 1 1 0],[0 0 1 1],c1);patch([0 1 1 1-e 1-e 0+e],[0 0 1 1-e 0+e 0+e],c2);patch([0 0 1 1-e 0+e 0+e],[0 1 1 1-e 1-e 0+e],c3);plot([0 1 1 0 0],[0 0 1 1 0]);disp('Mux')
  "pd{2,1}" : Outport
      mask Display: e = 0.06;c1 = [120 230 180]/255;c2 = ([120 230 180]+0)/(256+128);c3 = ([120 230 180]+128)/(256+128);patch([0 1 1 0],[0 0 1 1],c1);patch([0 1 1 1-e 1-e 0+e],[0 0 1 1-e 0+e 0+e],c2);patch([0 0 1 1-e 0+e 0+e],[0 1 1 1-e 1-e 0+e],c3);plot([0 1 1 0 0],[0 0 1 1 0]);
  wires:
  "p{2}"/1 -> mux/1
  mux/1 -> "pd{2,1}"/1
